simulink library "value"  (R2025b)
settings: Solver=VariableStepAuto  StartTime=0.0  StopTime=10.0  RelTol=1e-3
settings Model: Creator=ciepm  LastModifiedBy=aodha

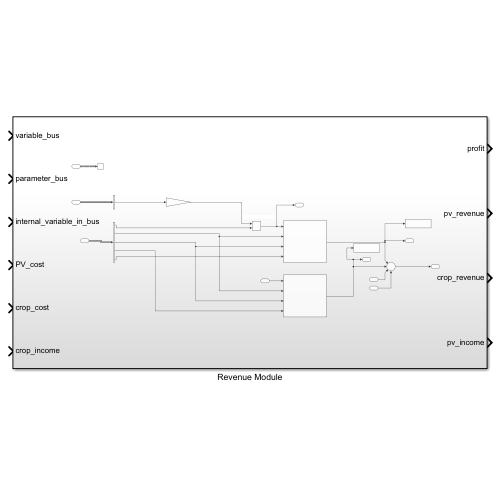
[thumbnail: Simulink's stored preview of the top-level diagram]
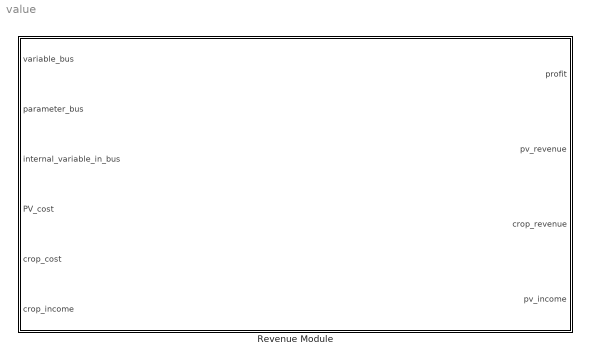
== system value ==
  Revenue Module : Subsystem

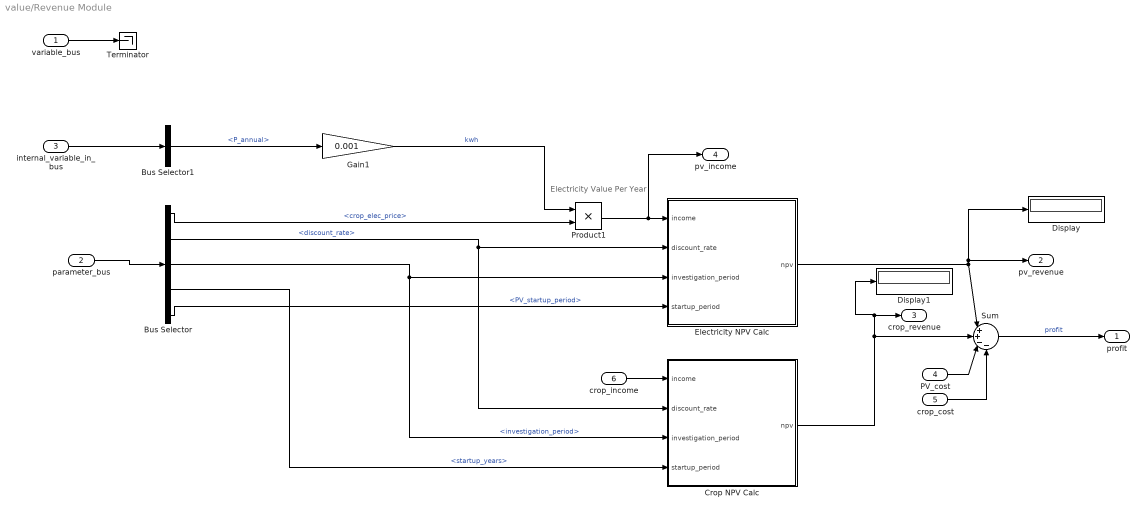
== system value/Revenue Module ==
  note: Electricity Value Per Year
  variable_bus : Inport
  parameter_bus : Inport  Port=2
  internal_variable_in_bus : Inport  Port=3
  PV_cost : Inport  Port=4
  crop_cost : Inport  Port=5
  crop_income : Inport  Port=6
  Bus Selector : BusSelector  OutputSignals=crop_elec_price,discount_rate,investigation_period,startup_years,PV_startup_period
  Bus Selector1 : BusSelector  OutputSignals=energy_per_year.P_annual
  Crop NPV Calc : MATLAB Function  TreatAsAtomicUnit=on
  Display : Display
  Display1 : Display
  Electricity NPV Calc : MATLAB Function  TreatAsAtomicUnit=on
  Gain1 : Gain  Gain=0.001
  Product1 : Product
  Sum : Sum  Inputs=|++--
  Terminator : Terminator
  profit : Outport
  pv_revenue : Outport  Port=2
  crop_revenue : Outport  Port=3
  pv_income : Outport  Port=4
  wires:
  Bus Selector/4 -> Crop NPV Calc/4(startup_period)  "<startup_years>"
  Bus Selector/5 -> Electricity NPV Calc/4(startup_period)  "<PV_startup_period>"
  Electricity NPV Calc/1(npv) -> Sum/1, pv_revenue/1, Display/1
  crop_income/1 -> Crop NPV Calc/1(income)
  Crop NPV Calc/1(npv) -> Sum/2, crop_revenue/1, Display1/1
  Bus Selector/3 -> Electricity NPV Calc/3(investigation_period), Crop NPV Calc/3(investigation_period)  "<investigation_period>"
  Bus Selector/2 -> Electricity NPV Calc/2(discount_rate), Crop NPV Calc/2(discount_rate)  "<discount_rate>"
  Product1/1 -> Electricity NPV Calc/1(income), pv_income/1
  Bus Selector/1 -> Product1/2  "<crop_elec_price>"
  variable_bus/1 -> Terminator/1
  crop_cost/1 -> Sum/4
  PV_cost/1 -> Sum/3
  Gain1/1 -> Product1/1  "kwh"
  Bus Selector1/1 -> Gain1/1  "<P_annual>"
  internal_variable_in_bus/1 -> Bus Selector1/1
  parameter_bus/1 -> Bus Selector/1
  Sum/1 -> profit/1  "profit"

== matlab function value/Revenue Module/Crop NPV Calc ==
  data: income input; npv output; discount_rate input; investigation_period input; startup_period input
function npv = calc_discounted_cash_flow(income, discount_rate, investigation_period,startup_period)
    exponent_value = startup_period:investigation_period-1;
    npv = sum(income ./ (1 + discount_rate).^exponent_value)+0.1.*(income./(1+discount_rate).^(startup_period-1));
end

== matlab function value/Revenue Module/Electricity NPV Calc ==
  data: income input; npv output; discount_rate input; investigation_period input; startup_period input
function npv = calc_discounted_cash_flow(income, discount_rate, investigation_period,startup_period)
    exponent_value = startup_period:investigation_period-1;
    npv = sum(income ./ (1 + discount_rate).^exponent_value);
end
